simulink model "range_estimaion"  (R2021a)
settings: Solver=VariableStepAuto  StartTime=0.0  StopTime=1220  RelTol=1e-3
undefined symbols (not defined in the file): DiscIntNeverNeededParam
libraries: qss_tb_library x5
settings Model: Creator=LENOVO  LastModifiedBy=LENOVO

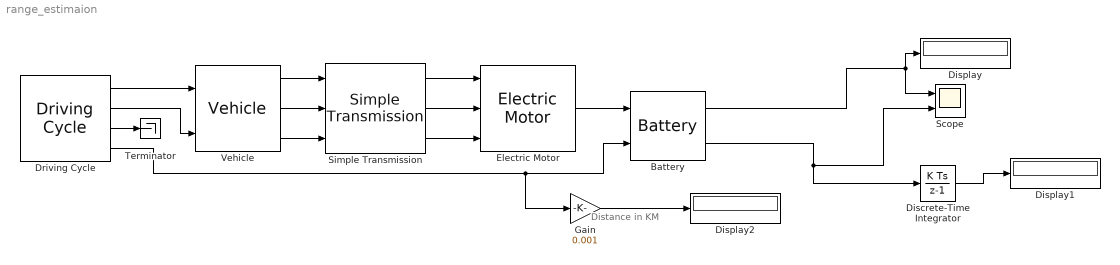
== system range_estimaion ==
  note: Distance in KM
  Battery : qss_tb_library/Energy Buffer/Battery  Tag=battery  I_0=150  Q_BT_IC_rel=80  t_ch=20
  Discrete-Time Integrator : DiscreteIntegrator  SampleTime=-1  ICPrevOutput=DiscIntNeverNeededParam  ICPrevScaledInput=DiscIntNeverNeededParam
  Display : Display
      settings: Decimation=2
  Display1 : Display
  Display2 : Display
  Driving Cycle : qss_tb_library/Driving Cycle/Driving Cycle  Tag=cycle  cyclenr=Europe: NEDC  stepsize=1  autostop=on
  Electric Motor : qss_tb_library/Energy Converter/Electric Motor  scale_EM=1  theta_EM=0.1  P_aux=0
  Gain : Gain  Gain=0.001
  Scope : Scope  NumInputPorts=2
  Simple Transmission : qss_tb_library/Gear System/Simple Transmission  Tag=simple transmission  gear_ratio=2  e_GT=0.98  P_GT0=50  w_wheel_min=1
  Terminator : Terminator
  Vehicle : qss_tb_library/Vehicle/Vehicle  Tag=vehicle  m_f=350  mt2m_f=5  A_f=1.5  d_wheel=0.3  cw=0.5  mu=0.015
  wires:
  Driving Cycle/1 -> Vehicle/1
  Driving Cycle/2 -> Vehicle/2
  Driving Cycle/4 -> Gain/1, Battery/2
  Driving Cycle/3 -> Terminator/1
  Vehicle/1 -> Simple Transmission/1
  Vehicle/2 -> Simple Transmission/2
  Vehicle/3 -> Simple Transmission/3
  Simple Transmission/1 -> Electric Motor/1
  Simple Transmission/2 -> Electric Motor/2
  Simple Transmission/3 -> Electric Motor/3
  Electric Motor/1 -> Battery/1
  Battery/1 -> Scope/1, Display/1
  Battery/2 -> Scope/2, Discrete-Time Integrator/1
  Discrete-Time Integrator/1 -> Display1/1
  Gain/1 -> Display2/1
